simulink model "MG2"  (R2020b)
settings: Solver=FixedStepAuto  StartTime=0.0  StopTime=TFinal  FixedStep=TDelay  RelTol=1e-3
undefined symbols (not defined in the file or in its folder): B, G, n, Nodes
libraries: simulink x1
settings Model: Creator=tian  LastModifiedBy=tian

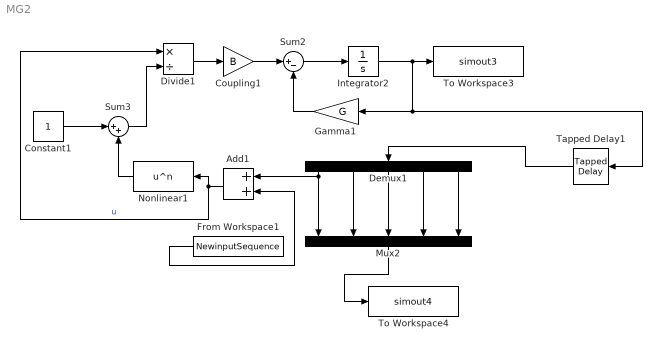
== system MG2 ==
  Add1 : Sum
  Constant1 : Constant
  Coupling1 : Gain  Gain=B
  Demux1 : Demux  Outputs=5
  Divide1 : Product  Inputs=*/
  From Workspace1 : FromWorkspace  VariableName=NewinputSequence
  Gamma1 : Gain  Gain=G
  Integrator2 : Integrator
  Mux2 : Mux  Inputs=5
  Nonlinear1 : Fcn  Expr=u^n
  Sum2 : Sum  Inputs=|+-
  Sum3 : Sum  Inputs=|++
  Tapped Delay1 : simulink/Discrete/Tapped Delay  vinit=0.0  samptime=TDelay  NumDelays=Nodes  DelayOrder=Oldest  includeCurrent=off
  To Workspace3 : ToWorkspace  VariableName=simout3  SampleTime=-1
      settings: Save2DSignal=2-D array (concatenate along first dimension)
  To Workspace4 : ToWorkspace  VariableName=simout4  SampleTime=-1
  wires:
  Divide1/1 -> Coupling1/1
  Coupling1/1 -> Sum2/1
  Tapped Delay1/1 -> Demux1/1
  Gamma1/1 -> Sum2/2
  Sum3/1 -> Divide1/2
  Add1/1 -> Divide1/1, Nonlinear1/1  "u"
  Nonlinear1/1 -> Sum3/2
  Sum2/1 -> Integrator2/1
  Integrator2/1 -> To Workspace3/1, Tapped Delay1/1, Gamma1/1
  Mux2/1 -> To Workspace4/1
  Constant1/1 -> Sum3/1
  Demux1/1 -> Mux2/1, Add1/1
  Demux1/2 -> Mux2/2
  Demux1/3 -> Mux2/3
  Demux1/4 -> Mux2/4
  Demux1/5 -> Mux2/5
  From Workspace1/1 -> Add1/2
